simulink model "Multicopter_vPC"  (R2021a)
settings: Solver=ode4  StartTime=0.0  StopTime=inf  FixedStep=0.0002  RelTol=1e-3
values from neighbouring files (symbols this model uses):
  ModelFailBatt_CustomHovTime = 15    [Init.m]
  ModelFailBatt_isEnable = boolean(0)    [Init.m]
  ModelFailBatt_islowCapacity = boolean(0)    [Init.m]
  ModelFailBatt_isLowVoltage = boolean(0)    [Init.m]
  ModelFailBatt_isPowOff = boolean(0)    [Init.m]
  ModelFailBatt_isUseCustomHovTime = boolean(0)    [Init.m]
  ModelFailBatt_remainCapacityRatio = 0.2    [Init.m]
  ModelFailBatt_remainVoltageRatio = 0.5    [Init.m]
  ModelFailEnable = boolean(0)    [Init.m]
  ModelFailLoad_isEnable = boolean(0)    [Init.m]
  ModelFailLoad_isLoadFall = boolean(0)    [Init.m]
  ModelFailLoad_isLoadLeak = boolean(0)    [Init.m]
  ModelFailLoad_isLoadShift = boolean(0)    [Init.m]
  ModelFailLoad_LoadLeakRatioRate = 0    [Init.m]
  ModelFailLoad_loadMassRatio = 0    [Init.m]
  ModelFailLoad_LoadShiftXRatio = 0    [Init.m]
  ModelFailLoad_LoadShiftYRatio = 0    [Init.m]
  ModelFailLoad_LoadShiftZRatio = 0    [Init.m]
  ModelFailProp_isEnable = boolean(1)    [Init.m]
  ModelFailProp_PropEffRatioVec = ones(1,8)    [Init.m]
  ModelFailWind_ConstWindX = 0    [Init.m]
  ModelFailWind_ConstWindY = 0    [Init.m]
  ModelFailWind_ConstWindZ = 0    [Init.m]
  ModelFailWind_GustWindFreq = 0    [Init.m]
  ModelFailWind_GustWindStrength = 0    [Init.m]
  ModelFailWind_isConstWind = boolean(0)    [Init.m]
  ModelFailWind_isEnable = boolean(0)    [Init.m]
  ModelFailWind_isGustWind = boolean(0)    [Init.m]
  ModelFailWind_isSheerWind = boolean(0)    [Init.m]
  ModelFailWind_isTurbWind = boolean(0)    [Init.m]
  ModelFailWind_SheerWindDirec = 0    [Init.m]
  ModelFailWind_SheerWindStrength = 0    [Init.m]
  ModelFailWind_TurbWindDirec = 0    [Init.m]
  ModelFailWind_TurbWindStrength = 0    [Init.m]
  ModelInit_RPM = 0    [Init.m]
  ModelParam_BattHoverMinutes = 18    [Init.m]
  ModelParam_BattHoverThr = 0.609    [Init.m]
  ModelParam_envAltitude = -41.5260009765625    (= -41.5260009766)    [Init.m]
  ModelParam_GlobalNoiseGainSwitch = 0    [Init.m]
  ModelParam_GPSEphFinal = 0.3    [Init.m]
  ModelParam_GPSEpvFinal = 0.4    [Init.m]
  ModelParam_GPSFix3DFix = 3    [Init.m]
  ModelParam_GPSSatsVisible = 10    [Init.m]
  ModelParam_motorCr = 1148    [Init.m]
  ModelParam_motorJm = 0.0001287    [Init.m]
  ModelParam_motorMinThr = 0.05    [Init.m]
  ModelParam_motorT = 0.02    [Init.m]
  ModelParam_motorWb = -141.4    [Init.m]
  ModelParam_noiseBaroCoupleWithSpeed = 0    [Init.m]
  ModelParam_noiseGPSSampTime = 0.2    [Init.m]
  ModelParam_noisePowerIMU = 0    [Init.m]
  ModelParam_noisePowerOffGainAccel = 0.04    [Init.m]
  ModelParam_noisePowerOffGainAccelZ = 0.03    [Init.m]
  ModelParam_noisePowerOffGainGyro = 0.02    [Init.m]
  ModelParam_noisePowerOffGainGyroZ = 0.025    [Init.m]
  ModelParam_noisePowerOffGainMag = 0.02    [Init.m]
  ModelParam_noisePowerOffGainMagZ = 0.035    [Init.m]
  ModelParam_noisePowerOnGainAccel = 0.8    [Init.m]
  ModelParam_noisePowerOnGainAccelZ = 4.5    [Init.m]
  ModelParam_noisePowerOnGainGyro = 2    [Init.m]
  ModelParam_noisePowerOnGainGyroZ = 1    [Init.m]
  ModelParam_noisePowerOnGainMag = 0.025    [Init.m]
  ModelParam_noisePowerOnGainMagZ = 0.05    [Init.m]
  ModelParam_noiseSampleTimeAccel = 0.001    [Init.m]
  ModelParam_noiseSampleTimeGyro = 0.001    [Init.m]
  ModelParam_noiseSampleTimeMag = 0.01    [Init.m]
  ModelParam_noiseUpperBaro = 0    [Init.m]
  ModelParam_noiseUpperGPS = 0.5    [Init.m]
  ModelParam_noiseUpperWindBodyRatio = 0    [Init.m]
  ModelParam_noiseWindSampTime = 0.001    [Init.m]
  ModelParam_rotorCm = 1.779e-07    [Init.m]
  ModelParam_rotorCt = 1.105e-05    [Init.m]
  ModelParam_timeSampBaro = 0.01    [Init.m]
  ModelParam_uavCCm = [0.0035 0.0039 0.0034]    [Init.m]
  ModelParam_uavCd = 0.055    [Init.m]
  ModelParam_uavDearo = 0.12    [Init.m]
  ModelParam_uavJ = [ModelParam_uavJxx,0,0;     0,ModelParam_uavJyy,0;     0,0,ModelParam_uavJzz]    [Init.m]
  ModelParam_uavMass = 1.4    [Init.m]
  ModelParam_uavMotNumbs = int8(4)    [Init.m]
  ModelParam_uavR = 0.225    [Init.m]
  ModelParam_uavType = int8(3)    [Init.m]
undefined symbols (not defined in the file or in its folder): d_i, Earth, F, h_i, Light, MIL, ModelParam_GPSEphInitial, ModelParam_GPSEphTimeConstant, ModelParam_GPSEpvInitial, ModelParam_GPSEpvTimeConstant, ModelParam_noiseLowPassFilterCoeAccel, ModelParam_noiseLowPassFilterCoeGyro, ModelParam_timeSamp, Moderate, Newton, Raphson, WGS84
libraries: simulink x12, aerolibasang x4, aerolibwind2 x3, aerolibtransform2 x3, sharedtransform x3, aerolibutil x2, sharedutil x2, shared6dof x1, aerolibatmos2 x1, aerolibconvert2 x1, aerolibobsolete x1, aerolibnav x1
(part 3 of 3)

== matlab function Multicopter_vPC/Actuator Model: Motor_ESC/Propeller Fail model ==
  data: u input; y output; isEnable input; PropEffRatioVec input
function y = fcn(u, isEnable, PropEffRatioVec)
% This is a propeller failure model. PropEffRatioVec is a 1*8 vector 
% about propeller efficiency with the value range [0 1]. 

if isEnable
    y=PropEffRatioVec.*u;
else
    y = u;    
end

== matlab function Multicopter_vPC/OutputPort/HILGPSModel/-pi-pi---->0-2pi ==
  data: yaw180 input; yaw360 output
function yaw360 = fcn(yaw180)
%//rad
if yaw180>0
    yaw360 = yaw180;
else
    yaw360 = yaw180 +2*pi;
end

== matlab function Multicopter_vPC/OutputPort/HILSensorMavModel/MATLAB Function ==
  data: h input; p output
function p = fcn(h)
p=((1-h/0.3048/145366.45))^(1/0.190284)*101325;

== matlab function Multicopter_vPC/OutputPort/HILGPSModel/GenCogVel ==
  data: v output; u input; cot output
function [v,cot] = Ang360(u)
 cot=atan2d(u(2),u(1));
if cot<0
    cot=cot+360;
end

v=norm(u(1:2));

== matlab function Multicopter_vPC/Environment Model/MATLAB Function ==
  settings: updateMethod=DISCRETE
  data: t input; isGustWind input; gWind output; GustWindStrength input; GustWindFreq input; turb input
function gWind = GustWindModel(t,isGustWind,GustWindStrength,GustWindFreq,turb)

if(GustWindFreq<1)
    GustWindFreq=1;
end
timeVel=60/GustWindFreq;

vmax=GustWindStrength;

persistent t0;
if isempty(t0)
    t0=0;
end

persistent isInGust;
if isempty(isInGust)
    isInGust=0;
end

persistent t1;
if isempty(t1)
    t1=2;
end

persistent a;
if isempty(a)
    a=0.5;
end

persistent ang;
if isempty(ang)
    ang=pi/2;
end

persistent wlast;
if isempty(wlast)
    wlast=vmax*0.5;
end

persistent wNow;
if isempty(wNow)
    wNow=1.4*0.8*vmax;
end


if isGustWind&&isInGust<0.5
    t0=t;
    t1=timeVel*(3/4+1/2*rand(1));
    a=1/4+1/2*rand(1);
    ang=pi*2*rand(1);
    wlast=wNow;
    wNow=1.2*(rand(1)*0.5+0.5)*vmax;
    
    isInGust=1;
end

if ~isGustWind
    isInGust=0;
end

gWind=[0;0;0];

if(t<t0+t1*a)
    gWindMag=(wNow-wlast)/2*(1-cos((t-t0)/(t1*a)*pi))+wlast;
else
    gWindMag=wNow;
end

if abs(t-(t0+t1))<0.05
    rng(t*1000);
    t0=t;
    t1=timeVel*(3/4+1/2*rand(1));
    a=1/4+1/2*rand(1);
    ang=ang+0.1*pi*rand(1);
    wlast=wNow;
    wNow=1.2*(rand(1)*0.5+0.5)*vmax;
end

gWind(1)=gWindMag*cos(ang)*0.8+turb(1)*0.4;
gWind(2)=gWindMag*sin(ang)*0.8+turb(2)*0.4;
gWind(3)=turb(3)*0.4;
